simulink model "filtro_media_movel_4"  (R2019b)
settings: Solver=VariableStepAuto  StartTime=0.0  StopTime=10.0  RelTol=1e-3
values from neighbouring files (symbols this model uses):
  T = 0.00833333333333    [ECG_graficos_fft.mat]    (also in FPB_Arduino.mat = 0.001; butter1.mat = 1.25e-08; filtro_notch1.mat; intro_resp_freq.mat = 0.00125)
settings Model: Creator=fernandopassold  LastModifiedBy=fernandopassold

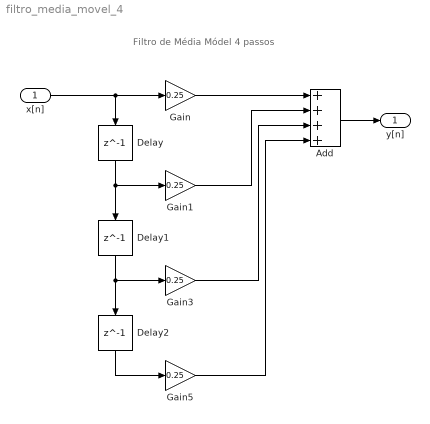
== system filtro_media_movel_4 ==
  note: Filtro de Média Módel
      | 4 passos
  x[n] : Inport
  Add : Sum  Inputs=++++
  Delay : Delay  DelayLength=1  SampleTime=T
  Delay1 : Delay  DelayLength=1  SampleTime=T
  Delay2 : Delay  DelayLength=1  SampleTime=T
  Gain{,1,3,5} (4 alike) : Gain  Gain=0.25
  y[n] : Outport
  wires:
  x[n]/1 -> Delay/1, Gain/1
  Delay/1 -> Delay1/1, Gain1/1
  Delay1/1 -> Delay2/1, Gain3/1
  Delay2/1 -> Gain5/1
  Gain/1 -> Add/1
  Gain1/1 -> Add/2
  Gain3/1 -> Add/3
  Gain5/1 -> Add/4
  Add/1 -> y[n]/1
